simulink model "SP_OEL"  (R2023b)
settings: Solver=VariableStepAuto  StartTime=0.0  StopTime=1  RelTol=1e-3
undefined symbols (not defined in the file or in its folder): relay1, relay2, source
libraries: ee_lib x31, fl_lib x16, eeGeneralControl x8, nesl_utility x7, simulink x4, simulink_extras x4, spspowerguiLib x1
(part 1 of 2)
settings Model: Creator=hazwani  LastModifiedBy=yeowy
settings ModelReferenceCC: EnableRefExpFcnMdlSchedulingChecks=on

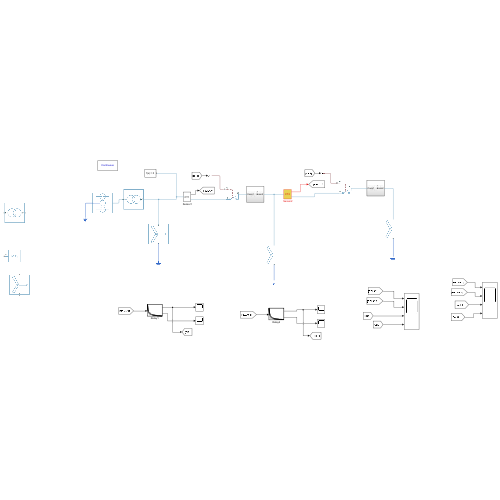
[thumbnail: Simulink's stored preview of the top-level diagram]
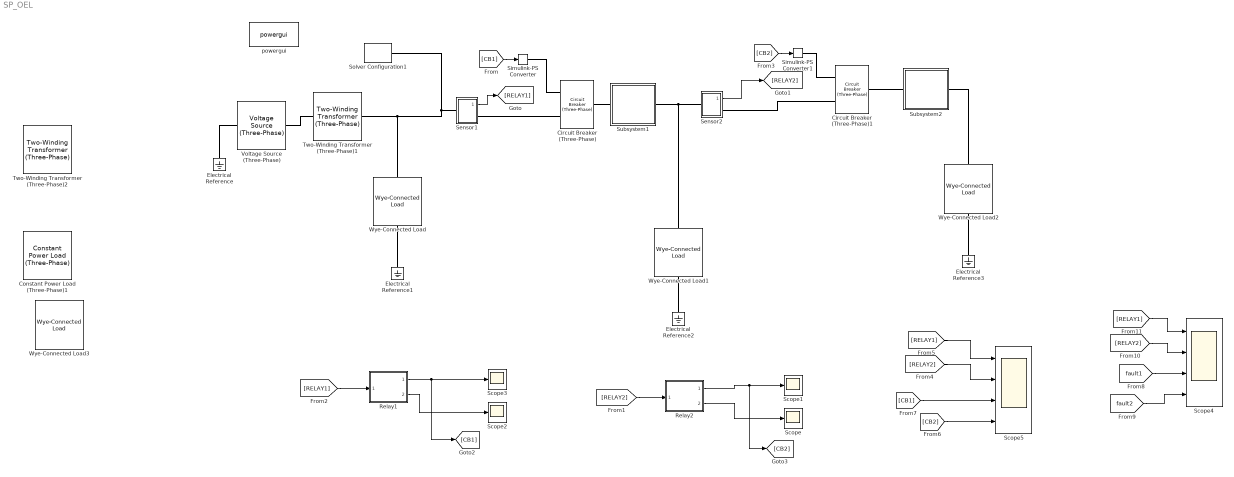
== system SP_OEL ==
  " Sensor1" : Subsystem
      mask Display: disp('CT1')
  " Sensor2" : Subsystem
      mask Display: disp('CT2')
  Circuit Breaker (Three-Phase) : ee_lib/Switches & Breakers/Circuit Breaker (Three-Phase)  R_closed=0.001 Ohm  G_open=1e-6 1/Ohm  threshold=11*(1./sqrt(3)) kV  breaker_behavior=ee.enum.switches.breakerBehavior.zeroCrossingEnable
      settings: InternalSimscapePortConfiguration="{\"Bottom\":[],\"Left\":[{\"id\":\"vT\",\"label\":\"vT\",\"type\":\"input\"},{\"id\":\"N1\",\"label\":\"~1\",\"type\":\"foundation.electrical.three_phase\"}],\"Right\":[{\"id\":\"N2\",\"label\":\"~2\",\"type\":\"foundation.electrical.three_phase\"}],\"Top\":[]}"
  Circuit Breaker (Three-Phase)1 : ee_lib/Switches & Breakers/Circuit Breaker (Three-Phase)  R_closed=0.001 Ohm  G_open=1e-6 1/Ohm  threshold=11*(1./sqrt(3)) kV  breaker_behavior=ee.enum.switches.breakerBehavior.zeroCrossingEnable
      settings: InternalSimscapePortConfiguration="{\"Bottom\":[],\"Left\":[{\"id\":\"vT\",\"label\":\"vT\",\"type\":\"input\"},{\"id\":\"N1\",\"label\":\"~1\",\"type\":\"foundation.electrical.three_phase\"}],\"Right\":[{\"id\":\"N2\",\"label\":\"~2\",\"type\":\"foundation.electrical.three_phase\"}],\"Top\":[]}"
  Constant Power Load (Three-Phase)1 : ee_lib/Passive/Constant Power Load (Three-Phase)  port_option=ee.enum.threePhasePort.composite  FRated=50 Hz  active_power=10 MW  reactive_power=4000 A*kV  Vline_rms_min=11 kV  tau=0.01 s  Vline_rms_ini=11 kV  Vang_ini=0 deg  gmin=1e-6 S  enable_fault=simscape.enum.onoff.off  fault_action=simscape.enum.assert.action.none  t_fault=1 s  open_conductance=1e-4 S
      settings: InternalSimscapePortConfiguration="{\"Bottom\":[],\"Left\":[{\"id\":\"N\",\"label\":\"~\",\"type\":\"foundation.electrical.three_phase\"}],\"Right\":[],\"Top\":[]}"
  Electrical Reference{,1..3} (4 alike) : fl_lib/Electrical/Electrical Elements/Electrical Reference
  Relay1 : Subsystem  TreatAsAtomicUnit=on  SystemSampleTime=relay1.sampleTime  mask{relayCharacteristicPhase=IEC Normal Inverse, relayCharacteristicEarth=IEC Normal Inverse, ratedFrequency=source.ratedFrequency, sampleTime=relay1.sampleTime, protectionEnable=1, currentPhase=[1.5 2.5 3.5 4.5 5.5 6.5 7.5 8.5 9.5 10.5], tmsPhase=[0.1 0.2], topPhase=[0.64 1.29;0.29 0.58;0.21 0.43;0.18 0.36;0.16 0.32;0.15 0.29;0.14 0.27;0.13 0.26;0.12 0.25;0.12 0.24], currentEarth=[0.06 0.15 0.2 0.25 0.3 0.35 0.4 0.45 0.5 0.55], tmsEarth=[0.1 0.2], topEarth=[0.64 1.29;0.29 0.58;0.21 0.43;0.18 0.36;0.16 0.32;0.15 0.29;0.14 0.27;0.13 0.26;0.12 0.25;0.12 0.24], phPickUp=relay1.phFltPickUp, ethPickUp=relay1.erFltPickUp, phTimeSetting=relay1.phFltTMS, ethTimeSetting=relay1.erFltTMS, topPhaseActual=0.2, topEarthActual=0.3}
      mask prompts: relayCharacteristicPhase "Relay characteristics for phase protection"; relayCharacteristicEarth "Relay characteristics for earth protection"; ratedFrequency "Fundamental frequency (Hz)"; sampleTime "Relay sample time (s)"; protectionEnable "Relay operation enable"; currentPhase "Current setting for phase protection (A)"; tmsPhase "Time multiplier setting for phase protection (s)"; topPhase "Operating time for phase protection (s)"; currentEarth "Current setting for earth protection (A)"; tmsEarth "Time multiplier setting for earth protection (s)"; topEarth "Operating time for earth protection (s)"; phPickUp "Pick up current for phase protection (A)"; ethPickUp "Pick up current for earth protection (A)"; phTimeSetting "Time multiplier setting for phase protection (s)"; ethTimeSetting "Time multiplier setting for earth protection (s)"; topPhaseActual "Relay operating time for phase protection (s)"; topEarthActual "Relay operating time for earth protection (s)"
      mask TypeOptions relayCharacteristicPhase: IEC Normal Inverse | IEC Very Inverse | IEC Extremely Inverse | IEEE Moderately Inverse | IEEE Very Inverse | IEEE Extremely Inverse | Definite Time | IvsT
      mask Callback relayCharacteristicPhase:
      | % Control parameter visiblity
      | enablePhase = get_param(gcb,'relayCharacteristicPhase');
      | enableEarth = get_param(gcb,'relayCharacteristicEarth');
      | % Set the 'MaskVisibilities' property for each parameters
      | cArray=cell(1,17);
      | cArray(:)={'on'};
      | p=strcmp(enablePhase,'IvsT');
      | q=strcmp(enableEarth,'IvsT');
      | r=strcmp(enablePhase,'Definite Time');
      | s=strcmp(enableEarth,'Definite Time');
      | if p==0 && q==1
      |     cArray(6:8)={'off'};
      | elseif p==0 && q==0
      |     cArray(6:11)={'off'};
      | elseif p==1 && q==0
      |     cArray(9:11)={'off'};
      | end
      | if r==0 && s==1
      |     cArray(15)={'off'};
      |     cArray(16)={'off'};
      | elseif r==0 && s==0
      |     cArray(16:17)={'off'};
      | elseif r==1 && s==0
      |     cArray(14)={'off'};
      |     cArray(17)={'off'};
      | elseif r==1 && s==1
      |     cArray(14:15)={'off'};
      | end
      | set_param(gcb,'MaskVisibilities',cArray);
      mask TypeOptions relayCharacteristicEarth: IEC Normal Inverse | IEC Very Inverse | IEC Extremely Inverse | IEEE Moderately Inverse | IEEE Very Inverse | IEEE Extremely Inverse | Definite Time | IvsT
      mask Callback relayCharacteristicEarth:
      | % Control parameter visiblity
      | enablePhase = get_param(gcb,'relayCharacteristicPhase');
      | enableEarth = get_param(gcb,'relayCharacteristicEarth');
      | % Set the 'MaskVisibilities' property for each parameters
      | cArray=cell(1,17);
      | cArray(:)={'on'};
      | p=strcmp(enablePhase,'IvsT');
      | q=strcmp(enableEarth,'IvsT');
      | r=strcmp(enablePhase,'Definite Time');
      | s=strcmp(enableEarth,'Definite Time');
      | if p==0 && q==1
      |     cArray(6:8)={'off'};
      | elseif p==0 && q==0
      |     cArray(6:11)={'off'};
      | elseif p==1 && q==0
      |     cArray(9:11)={'off'};
      | end
      | if r==0 && s==1
      |     cArray(15)={'off'};
      |     cArray(16)={'off'};
      | elseif r==0 && s==0
      |     cArray(16:17)={'off'};
      | elseif r==1 && s==0
      |     cArray(14)={'off'};
      |     cArray(17)={'off'};
      | elseif r==1 && s==1
      |     cArray(14:15)={'off'};
      | end
      | set_param(gcb,'MaskVisibilities',cArray);
      mask DialogControl Container9 Prompt: Main
      mask DialogControl Container24 Prompt: Current Settings
      mask DialogControl Container19 Prompt: Time Settings
      mask Display:
      | psm = 1:1:30; % Plug setting multiplier
      | tms=0.01; % Time multiplier setting is assumed to be 0.01s
      | top=ones(2,length(psm));  % Operating time of the relay
      | maskParameter=Simulink.Mask.get(gcb); % Get the mask parameters
      | for i=1:2
      |     index(i)=find(strcmp(maskParameter.Parameters(1,i).Value,maskParameter.Parameters(1,i).TypeOptions));
      |     if index(i)<7
      |         switch index(i)              % Selection of relay characteristic
      |             case 1                   % IEC Normal Inverse
      |                 a=0.14;
      |                 b=0.02;
      |                 c=0;
      |             case 2                   % IEC Very Inverse
      |                 a=13.5;
      |                 b=1;
      |                 c=0;
      |             case 3                   % IEC Extremely Inverse
      |                 a=80;
      |                 b=2;
      |                 c=0;
      |             case 4                   % IEEE Moderately Inverse
      |                 a=0.0515;
      |                 b=0.02;
      |                 c=0.114;
      |             case 5                   % IEEE Very Inverse
      |                 a=19.61;
      |                 b=2;
      |                 c=0.491;
      |             otherwise                % IEEE Exteremely Inverse
      |                 a=28.2;
      |                 b=2;
      |                 c=0.1217;
      |         end
      |         for j=1:length(psm)
      |             top(i,j)=tms*((a/(power(psm(j),b)-1))+c); % Operating time of the relay
      |         end
      |     else
      |         top(i,1:length(psm))=0.03*ones(1,length(psm));% Operating time of the relay
      |     end
      | end
      | top1=top(1,1:end);
      | top2=top(2,1:end);
      | 
      | maskFigure=figure;
      | if index(1)<8
      |     plot(psm,top1)
      | else
      |     fprintf('\n\nIvsT');
      | end
      | hold on;
      | if index(2)<8
      |     plot(psm,top2);
      | elseif index(1)<8
      |     fprintf('\nIvsT');
      | end
      | close(maskFigure);
  Relay2 : Subsystem  TreatAsAtomicUnit=on  SystemSampleTime=relay1.sampleTime  mask{relayCharacteristicPhase=IEEE Moderately Inverse, relayCharacteristicEarth=IEEE Moderately Inverse, ratedFrequency=source.ratedFrequency, sampleTime=relay2.sampleTime, protectionEnable=1, currentPhase=[1.5 2.5 3.5 4.5 5.5 6.5 7.5 8.5 9.5 10.5], tmsPhase=[0.1 0.2], topPhase=[0.64 1.29;0.29 0.58;0.21 0.43;0.18 0.36;0.16 0.32;0.15 0.29;0.14 0.27;0.13 0.26;0.12 0.25;0.12 0.24], currentEarth=[0.06 0.15 0.2 0.25 0.3 0.35 0.4 0.45 0.5 0.55], tmsEarth=[0.1 0.2], topEarth=[0.64 1.29;0.29 0.58;0.21 0.43;0.18 0.36;0.16 0.32;0.15 0.29;0.14 0.27;0.13 0.26;0.12 0.25;0.12 0.24], phPickUp=relay2.phFltPickUp, ethPickUp=relay2.erFltPickUp, phTimeSetting=relay2.phFltTMS, ethTimeSetting=relay2.erFltTMS, topPhaseActual=0.2, topEarthActual=0.3}
      mask prompts: relayCharacteristicPhase "Relay characteristics for phase protection"; relayCharacteristicEarth "Relay characteristics for earth protection"; ratedFrequency "Fundamental frequency (Hz)"; sampleTime "Relay sample time (s)"; protectionEnable "Relay operation enable"; currentPhase "Current setting for phase protection (A)"; tmsPhase "Time multiplier setting for phase protection (s)"; topPhase "Operating time for phase protection (s)"; currentEarth "Current setting for earth protection (A)"; tmsEarth "Time multiplier setting for earth protection (s)"; topEarth "Operating time for earth protection (s)"; phPickUp "Pick up current for phase protection (A)"; ethPickUp "Pick up current for earth protection (A)"; phTimeSetting "Time multiplier setting for phase protection (s)"; ethTimeSetting "Time multiplier setting for earth protection (s)"; topPhaseActual "Relay operating time for phase protection (s)"; topEarthActual "Relay operating time for earth protection (s)"
      mask TypeOptions relayCharacteristicPhase: IEC Normal Inverse | IEC Very Inverse | IEC Extremely Inverse | IEEE Moderately Inverse | IEEE Very Inverse | IEEE Extremely Inverse | Definite Time | IvsT
      mask Callback relayCharacteristicPhase:
      | % Control parameter visiblity
      | enablePhase = get_param(gcb,'relayCharacteristicPhase');
      | enableEarth = get_param(gcb,'relayCharacteristicEarth');
      | % Set the 'MaskVisibilities' property for each parameters
      | cArray=cell(1,17);
      | cArray(:)={'on'};
      | p=strcmp(enablePhase,'IvsT');
      | q=strcmp(enableEarth,'IvsT');
      | r=strcmp(enablePhase,'Definite Time');
      | s=strcmp(enableEarth,'Definite Time');
      | if p==0 && q==1
      |     cArray(6:8)={'off'};
      | elseif p==0 && q==0
      |     cArray(6:11)={'off'};
      | elseif p==1 && q==0
      |     cArray(9:11)={'off'};
      | end
      | if r==0 && s==1
      |     cArray(15)={'off'};
      |     cArray(16)={'off'};
      | elseif r==0 && s==0
      |     cArray(16:17)={'off'};
      | elseif r==1 && s==0
      |     cArray(14)={'off'};
      |     cArray(17)={'off'};
      | elseif r==1 && s==1
      |     cArray(14:15)={'off'};
      | end
      | set_param(gcb,'MaskVisibilities',cArray);
      mask TypeOptions relayCharacteristicEarth: IEC Normal Inverse | IEC Very Inverse | IEC Extremely Inverse | IEEE Moderately Inverse | IEEE Very Inverse | IEEE Extremely Inverse | Definite Time | IvsT
      mask Callback relayCharacteristicEarth:
      | % Control parameter visiblity
      | enablePhase = get_param(gcb,'relayCharacteristicPhase');
      | enableEarth = get_param(gcb,'relayCharacteristicEarth');
      | % Set the 'MaskVisibilities' property for each parameters
      | cArray=cell(1,17);
      | cArray(:)={'on'};
      | p=strcmp(enablePhase,'IvsT');
      | q=strcmp(enableEarth,'IvsT');
      | r=strcmp(enablePhase,'Definite Time');
      | s=strcmp(enableEarth,'Definite Time');
      | if p==0 && q==1
      |     cArray(6:8)={'off'};
      | elseif p==0 && q==0
      |     cArray(6:11)={'off'};
      | elseif p==1 && q==0
      |     cArray(9:11)={'off'};
      | end
      | if r==0 && s==1
      |     cArray(15)={'off'};
      |     cArray(16)={'off'};
      | elseif r==0 && s==0
      |     cArray(16:17)={'off'};
      | elseif r==1 && s==0
      |     cArray(14)={'off'};
      |     cArray(17)={'off'};
      | elseif r==1 && s==1
      |     cArray(14:15)={'off'};
      | end
      | set_param(gcb,'MaskVisibilities',cArray);
      mask DialogControl Container9 Prompt: Main
      mask DialogControl Container24 Prompt: Current Settings
      mask DialogControl Container19 Prompt: Time Settings
      mask Display:
      | psm = 1:1:30; % Plug setting multiplier
      | tms=0.01; % Time multiplier setting is assumed to be 0.01s
      | top=ones(2,length(psm));  % Operating time of the relay
      | maskParameter=Simulink.Mask.get(gcb); % Get the mask parameters
      | for i=1:2
      |     index(i)=find(strcmp(maskParameter.Parameters(1,i).Value,maskParameter.Parameters(1,i).TypeOptions));
      |     if index(i)<7
      |         switch index(i)              % Selection of relay characteristic
      |             case 1                   % IEC Normal Inverse
      |                 a=0.14;
      |                 b=0.02;
      |                 c=0;
      |             case 2                   % IEC Very Inverse
      |                 a=13.5;
      |                 b=1;
      |                 c=0;
      |             case 3                   % IEC Extremely Inverse
      |                 a=80;
      |                 b=2;
      |                 c=0;
      |             case 4                   % IEEE Moderately Inverse
      |                 a=0.0515;
      |                 b=0.02;
      |                 c=0.114;
      |             case 5                   % IEEE Very Inverse
      |                 a=19.61;
      |                 b=2;
      |                 c=0.491;
      |             otherwise                % IEEE Exteremely Inverse
      |                 a=28.2;
      |                 b=2;
      |                 c=0.1217;
      |         end
      |         for j=1:length(psm)
      |             top(i,j)=tms*((a/(power(psm(j),b)-1))+c); % Operating time of the relay
      |         end
      |     else
      |         top(i,1:length(psm))=0.03*ones(1,length(psm));% Operating time of the relay
      |     end
      | end
      | top1=top(1,1:end);
      | top2=top(2,1:end);
      | 
      | maskFigure=figure;
      | if index(1)<8
      |     plot(psm,top1)
      | else
      |     fprintf('\n\nIvsT');
      | end
      | hold on;
      | if index(2)<8
      |     plot(psm,top2);
      | elseif index(1)<8
      |     fprintf('\nIvsT');
      | end
      | close(maskFigure);
  Scope{,1..3} (4 alike) : Scope
  Scope4 : Scope  NumInputPorts=4
  Scope5 : Scope  NumInputPorts=4
  Simulink-PS Converter : nesl_utility/Simulink-PS Converter  PhysicalDomain=network_engine_domain  SubClassName=ps_input  LeftPortType=input  RightPortType=output  PseudoPeriodic=off  Frequencies=[]  NoiseDistribution=none  NoiseParameters=[]  Unit=1  AffineConversion=off  FilteringAndDerivatives=provide  SimscapeFilterOrder=1  InputFilterTimeConstant=0.001  UdotUserProvided=0
  Simulink-PS Converter1 : nesl_utility/Simulink-PS Converter  PhysicalDomain=network_engine_domain  SubClassName=ps_input  LeftPortType=input  RightPortType=output  PseudoPeriodic=off  Frequencies=[]  NoiseDistribution=none  NoiseParameters=[]  Unit=1  AffineConversion=off  FilteringAndDerivatives=provide  SimscapeFilterOrder=1  InputFilterTimeConstant=0.001  UdotUserProvided=0
  Solver Configuration1 : nesl_utility/Solver Configuration  PhysicalDomain=network_engine_domain  SubClassName=solver  LeftPortType=input  RightPortType=generic  Tones=[]  Harmonics=[]  SimulateNoise=off  Profile=off  UseLocalSampling=off  EnableSwitchedLinearOptims=on  FrequencyDomain=off  UseCCode=off  RelTol=0.001  AbsTol=0.001  MinStep=1e-09  ToWorkspace=off  RevertToSquareIcSolve=off  NumHomotopyIterations=100  PhasorMode=off  PhasorModeNumHarmonics=1  ConsistencySolver=NEWTON_XTOL_AFTER_FTOL  IndexReductionMethod=DerivativeReplacement  DoDC=on  ResidualTolerance=1e-09  ConsistencyTolSource=LOCAL  ConsistencyAbsTol=0.001  ConsistencyRelTol=0.001  ConsistencyTolFactor=0.001  UseLocalSolver=on  LocalSolverChoice=NE_TRAPEZOIDAL_ADVANCER  ResolveIndetEquations=on  FunctionEvalNumThread=1  LocalSolverSampleTime=0.001  DoFixedCost=on  MaxNonlinIter=3  MaxModeIter=2  ComputeImpulses=off  ImpulseIterations=2  LinearAlgebra=auto  LinearAlgebraNumThread=0  EquationFormulation=NE_TIME_EF  DelaysMemoryBudget=1024  AutomaticFiltering=on  FilteringTimeConstant=0.001  PartitionStorageMethod=AS_NEEDED  PartitionMemoryBudget=1024  PartitionMethod=ROBUST  MultibodyUseLocalSolver=off  MultibodyLocalSolverChoice=ODE1  MultibodyLocalSolverSampleTime=0.001
  Subsystem1 : Subsystem
  Subsystem2 : Subsystem
  Two-Winding Transformer (Three-Phase)1 : ee_lib/Passive/Transformers/Two-Winding Transformer (Three-Phase)  SRated=60e6 A*V  FRated=50 Hz  Winding1Connection=ee.enum.windingconnection.delta1  VRated1=33*(1./sqrt(3)) kV  Winding2Connection=ee.enum.windingconnection.Y  VRated2=11*(1./sqrt(3)) kV  CoreType=ee.enum.coretype.fivelimb  pu_Rw1=0.0014  pu_Rw2=0.0014  leakage_reactance_option=ee.enum.transformer_leakage.include  pu_Xl1=0.0624  pu_Xl2=0.0624  magnetizing_resistance_option=ee.enum.transformer_magnetizingResistance.include  pu_Rm=450  magnetizing_reactance_option=ee.enum.transformer_magnetizingReactance.include  saturation_option=ee.enum.transformer_saturation.exclude  pu_Xm=450  current_data=[0, .002, 1, 2]  magnetic_flux_data=[0, 1.2, 1.5, 1.51]  pu_X0=0.5  i1_specify=off  i1_priority=None  i1=[0, 0, 0] A  i1_nominal_specify=off  i1_nominal_unit=A  i1_nominal_value=1  i2_specify=off  i2_priority=None  i2=[0, 0, 0] A  i2_nominal_specify=off  i2_nominal_unit=A  i2_nominal_value=1  phi_specify=off  phi_priority=None  phi=[0, 0, 0]  phi_nominal_specify=off  phi_nominal_unit=1  phi_nominal_value=1  power_dissipated_specify=off  power_dissipated_priority=None  power_dissipated=0 W  power_dissipated_nominal_specify=off  power_dissipated_nominal_unit=W  power_dissipated_nominal_value=1
      settings: InternalSimscapePortConfiguration="{\"Bottom\":[],\"Left\":[{\"id\":\"N1\",\"label\":\"~1\",\"type\":\"foundation.electrical.three_phase\"}],\"Right\":[{\"id\":\"N2\",\"label\":\"~2\",\"type\":\"foundation.electrical.three_phase\"}],\"Top\":[]}"
  Two-Winding Transformer (Three-Phase)2 : ee_lib/Passive/Transformers/Two-Winding Transformer (Three-Phase)  SRated=60e6 A*V  FRated=50 Hz  Winding1Connection=ee.enum.windingconnection.delta1  VRated1=33*(1./sqrt(3)) kV  Winding2Connection=ee.enum.windingconnection.Y  VRated2=11*(1./sqrt(3)) kV  CoreType=ee.enum.coretype.fivelimb  pu_Rw1=0.0014  pu_Rw2=0.0014  leakage_reactance_option=ee.enum.transformer_leakage.include  pu_Xl1=0.0624  pu_Xl2=0.0624  magnetizing_resistance_option=ee.enum.transformer_magnetizingResistance.include  pu_Rm=450  magnetizing_reactance_option=ee.enum.transformer_magnetizingReactance.include  saturation_option=ee.enum.transformer_saturation.exclude  pu_Xm=450  current_data=[0, .002, 1, 2]  magnetic_flux_data=[0, 1.2, 1.5, 1.51]  pu_X0=0.5  i1_specify=off  i1_priority=None  i1=[0, 0, 0] A  i1_nominal_specify=off  i1_nominal_unit=A  i1_nominal_value=1  i2_specify=off  i2_priority=None  i2=[0, 0, 0] A  i2_nominal_specify=off  i2_nominal_unit=A  i2_nominal_value=1  phi_specify=off  phi_priority=None  phi=[0, 0, 0]  phi_nominal_specify=off  phi_nominal_unit=1  phi_nominal_value=1  power_dissipated_specify=off  power_dissipated_priority=None  power_dissipated=0 W  power_dissipated_nominal_specify=off  power_dissipated_nominal_unit=W  power_dissipated_nominal_value=1
      settings: InternalSimscapePortConfiguration="{\"Bottom\":[],\"Left\":[{\"id\":\"N1\",\"label\":\"~1\",\"type\":\"foundation.electrical.three_phase\"}],\"Right\":[{\"id\":\"N2\",\"label\":\"~2\",\"type\":\"foundation.electrical.three_phase\"}],\"Top\":[]}"
  Voltage Source (Three-Phase) : ee_lib/Sources/Voltage Source (Three-Phase)  vline_rms=33*(1./sqrt(3)) kV  shift=0 deg  freq=50 Hz  impedance_option=1  SShortCircuit=800e6 A*V  XR=5  R=0.01 Ohm  L=3.97e-4 H  harmonic_option=0  harmonic_orders=[5, 7, 11, 13]  harmonic_ratios=[.1, .1, .1, .1]  G_parasitic=0 1/Ohm  I_specify=off  I_priority=None  I=[0, 0, 0] A  I_nominal_specify=off  I_nominal_unit=A  I_nominal_value=1
  Wye-Connected Load : ee_lib/Passive/RLC Assemblies/Wye-Connected Load  parameterization=ee.enum.rlc.parameterization.ratedpower  component_structure=ee.enum.rlc.structure.R  component_structure_PQ=ee.enum.rlc.structure.SeriesRL  R=1 Ohm  L=1e-3 H  C=1e-6 F  VRated=11*(1./sqrt(3)) kV  FRated=50 Hz  P=10 MW  Qpos=4e6 A*V  Qneg=-1e2 A*V  R_parasitic=0 Ohm  G_parasitic=0 1/Ohm  R_parasitic_PQ=0 Ohm  G_parasitic_PQ=1e-6 1/Ohm  Vmag0=11*(1./sqrt(3)) kV  Vang0=0 deg  Freq0=50 Hz  IL_specify=off  IL_priority=High  IL=[0, 0, 0] A  IL_nominal_specify=off  IL_nominal_unit=A  IL_nominal_value=1  VC_specify=off  VC_priority=High  VC=[0, 0, 0] V  VC_nominal_specify=off  VC_nominal_unit=V  VC_nominal_value=1
  Wye-Connected Load1 : ee_lib/Passive/RLC Assemblies/Wye-Connected Load  parameterization=ee.enum.rlc.parameterization.ratedpower  component_structure=ee.enum.rlc.structure.R  component_structure_PQ=ee.enum.rlc.structure.SeriesRL  R=1 Ohm  L=1e-3 H  C=1e-6 F  VRated=11*(1./sqrt(3)) kV  FRated=50 Hz  P=10 MW  Qpos=4e6 A*V  Qneg=-1e2 A*V  R_parasitic=0 Ohm  G_parasitic=0 1/Ohm  R_parasitic_PQ=0 Ohm  G_parasitic_PQ=1e-6 1/Ohm  Vmag0=11*(1./sqrt(3)) kV  Vang0=0 deg  Freq0=50 Hz  IL_specify=off  IL_priority=High  IL=[0, 0, 0] A  IL_nominal_specify=off  IL_nominal_unit=A  IL_nominal_value=1  VC_specify=off  VC_priority=High  VC=[0, 0, 0] V  VC_nominal_specify=off  VC_nominal_unit=V  VC_nominal_value=1
  Wye-Connected Load2 : ee_lib/Passive/RLC Assemblies/Wye-Connected Load  parameterization=ee.enum.rlc.parameterization.ratedpower  component_structure=ee.enum.rlc.structure.R  component_structure_PQ=ee.enum.rlc.structure.SeriesRL  R=1 Ohm  L=1e-3 H  C=1e-6 F  VRated=11*(1./sqrt(3)) kV  FRated=50 Hz  P=20 MW  Qpos=10e6 A*V  Qneg=-1e2 A*V  R_parasitic=0 Ohm  G_parasitic=0 1/Ohm  R_parasitic_PQ=0 Ohm  G_parasitic_PQ=1e-6 1/Ohm  Vmag0=11*(1./sqrt(3)) kV  Vang0=0 deg  Freq0=50 Hz  IL_specify=off  IL_priority=High  IL=[0, 0, 0] A  IL_nominal_specify=off  IL_nominal_unit=A  IL_nominal_value=1  VC_specify=off  VC_priority=High  VC=[0, 0, 0] V  VC_nominal_specify=off  VC_nominal_unit=V  VC_nominal_value=1
  Wye-Connected Load3 : ee_lib/Passive/RLC Assemblies/Wye-Connected Load  parameterization=ee.enum.rlc.parameterization.ratedpower  component_structure=ee.enum.rlc.structure.R  component_structure_PQ=ee.enum.rlc.structure.SeriesRL  R=1 Ohm  L=1e-3 H  C=1e-6 F  VRated=11*(1./sqrt(3)) kV  FRated=50 Hz  P=10 MW  Qpos=4e6 A*V  Qneg=-1e2 A*V  R_parasitic=0 Ohm  G_parasitic=0 1/Ohm  R_parasitic_PQ=0 Ohm  G_parasitic_PQ=1e-6 1/Ohm  Vmag0=24e3 V  Vang0=0 deg  Freq0=60 Hz  IL_specify=off  IL_priority=High  IL=[0, 0, 0] A  IL_nominal_specify=off  IL_nominal_unit=A  IL_nominal_value=1  VC_specify=off  VC_priority=High  VC=[0, 0, 0] V  VC_nominal_specify=off  VC_nominal_unit=V  VC_nominal_value=1
  powergui : spspowerguiLib/powergui  Priority=1  SimulationMode=Continuous  SampleTime=50e-6  frequency=60  Iterations=50  frequencyindice=60  Pbase=100e6  ErrMax=1e-4  UnitsV=kV  UnitsW=MW  buscounter=0  FunctionMessages=off  echomessages=off  EnableUseOfTLC=off  CurrentSourceSwitches=off  DisableSnubberDevices=off  DisableRonSwitches=off  DisableVfSwitches=off  DisplayEquations=off  AutomaticDiscreteSolvers=off  SolverType=Tustin/Backward Euler (TBE)  Interpol=off  ExternalGateDelay=off  methode=off  Ts=100  x0status=blocks  SPID=on  SwTol=0  HookPort=off  NonlinearTolerance=1e-4  nMaxIteration=100  ContinueOnMaxIteration=off  RestoreLinks=warning  ResistiveCurrentMeasurement=off  Frange=[0:2:500]  Ylog=off  Xlog=on  ShowGrid=off  save=off  variable=ZData  structure=0  ZoomFFT=off  StartTime=0.0  cycles=1  DisplayStyle=1  fundamental=60  FreqAxis=off  MaxFrequency=1000  frequencyindicesteady=1  RmsSteady=1  display=off
  wires:
  " Sensor1"/1(Out1) -> [RELAY1]
  Relay2/2(Relay Status) -> Scope/1
  Relay2/1(Trip Signal) -> [CB2], Scope1/1
  Relay1/1(Trip Signal) -> [CB1], Scope3/1
  " Sensor2"/1(Out1) -> [RELAY2]
  [CB1] -> Simulink-PS Converter/1
  [CB2] -> Simulink-PS Converter1/1
  [RELAY2] -> Relay2/1(Inport)
  [RELAY1] -> Relay1/1(Inport)
  Relay1/2(Relay Status) -> Scope2/1
  [RELAY2] -> Scope5/2
  [RELAY1] -> Scope5/1
  [CB1] -> Scope5/3
  [CB2] -> Scope5/4
  [RELAY1] -> Scope4/1
  [RELAY2] -> Scope4/2
  [fault1] -> Scope4/3
  [fault2] -> Scope4/4
  connections:
  Voltage Source (Three-Phase)/LConn1 -- Electrical Reference/LConn1
  Two-Winding Transformer (Three-Phase)1/LConn1 -- Voltage Source (Three-Phase)/RConn1
  Electrical Reference1/LConn1 -- Wye-Connected Load/RConn1
  Solver Configuration1/RConn1 -- Two-Winding Transformer (Three-Phase)1/RConn1 -- Wye-Connected Load/LConn1 -- " Sensor1"/LConn1
  " Sensor1"/RConn1 -- Circuit Breaker (Three-Phase)/LConn2
  Circuit Breaker (Three-Phase)/RConn1 -- Subsystem1/LConn1
  Simulink-PS Converter/RConn1 -- Circuit Breaker (Three-Phase)/LConn1
  Circuit Breaker (Three-Phase)1/LConn1 -- Simulink-PS Converter1/RConn1
  Circuit Breaker (Three-Phase)1/RConn1 -- Subsystem2/LConn1
  Subsystem1/RConn1 -- Wye-Connected Load1/LConn1 -- " Sensor2"/LConn1
  Circuit Breaker (Three-Phase)1/LConn2 -- " Sensor2"/RConn1
  Wye-Connected Load1/RConn1 -- Electrical Reference2/LConn1
  Electrical Reference3/LConn1 -- Wye-Connected Load2/RConn1
  Wye-Connected Load2/LConn1 -- Subsystem2/RConn1

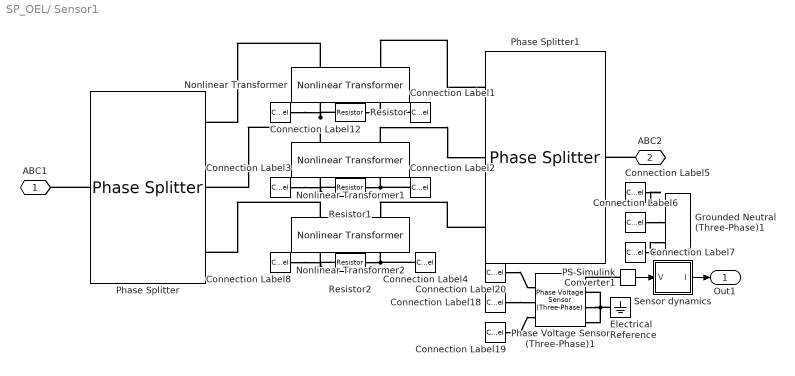
== system SP_OEL/ Sensor1 ==
  Connection Label1 : ConnectionLabel  Label=Ian
  Connection Label12 : ConnectionLabel  Label=Iap
  Connection Label18 : ConnectionLabel  Label=Ibp
  Connection Label19 : ConnectionLabel  Label=Icp
  Connection Label2 : ConnectionLabel  Label=Ibn
  Connection Label20 : ConnectionLabel  Label=Iap
  Connection Label3 : ConnectionLabel  Label=Ibp
  Connection Label4 : ConnectionLabel  Label=Ibn
  Connection Label5 : ConnectionLabel  Label=Ian
  Connection Label6 : ConnectionLabel  Label=Ibn
  Connection Label7 : ConnectionLabel  Label=Icn
  Connection Label8 : ConnectionLabel  Label=Icp
  Electrical Reference : fl_lib/Electrical/Electrical Elements/Electrical Reference
  Grounded Neutral (Three-Phase)1 : ee_lib/Connectors & References/Grounded Neutral (Three-Phase)
      settings: InternalSimscapePortConfiguration="{\"Bottom\":[],\"Left\":[{\"id\":\"a\",\"label\":\"a\",\"type\":\"foundation.electrical.electrical\"},{\"id\":\"b\",\"label\":\"b\",\"type\":\"foundation.electrical.electrical\"},{\"id\":\"c\",\"label\":\"c\",\"type\":\"foundation.electrical.electrical\"}],\"Right\":[],\"Top\":[]}"
  Nonlinear Transformer : ee_lib/Passive/Transformers/Nonlinear Transformer  Nw=1  Nw2=sensor1.ctRatio  winding_param_option=1  Req=1e-3 Ohm  Leq=1e-4 H  R_1=0.01 Ohm  L_1=0.0001 H  R_2=0.01 Ohm  L_2=0.0001 H  averaging_period=0 s  R_m=100 Ohm  parameterization_option=1  H_data=[0, 200, 400, 600, 800, 1000] A/m  B_data=[0, .81, 1.25, 1.42, 1.48, 1.49] T  length_effective=0.2 m  area_effective=2e-4 m^2  L=4e-2 H  L_sat=1e-2 H  current_data=[0, .4, .8, 1.2, 1.6, 2] A  magnetic_flux_data=[0, .161, .25, .284, .295, .299] .* 1e-3 Wb  magnetic_flux_sat=1.6e-04 Wb  dBdH0=0.005 m*T/A  B1=1.49 T  H1=1000 A/m  c=0.1  K=200 A/m  alpha=1e-4  interpolation_option=1  Leq_i0=0 A  L1_i0=0 A  L2_i0=0 A  x0_option=1  i_L0=0 A  phi0=0 Wb  B0=0 T  H0=0 A/m  Leq_g=1e-9 1/Ohm  L1_g=1e-9 1/Ohm  L2_g=1e-9 1/Ohm
      settings: InternalSimscapePortConfiguration="{\"Bottom\":[],\"Left\":[{\"id\":\"p1\",\"label\":\"1+\",\"type\":\"foundation.electrical.electrical\"},{\"id\":\"n1\",\"label\":\"1-\",\"type\":\"foundation.electrical.electrical\"}],\"Right\":[{\"id\":\"p2\",\"label\":\"2+\",\"type\":\"foundation.electrical.electrical\"},{\"id\":\"n2\",\"label\":\"2-\",\"type\":\"foundation.electrical.electrical\"}],\"Top\":[]}"
  Nonlinear Transformer1 : ee_lib/Passive/Transformers/Nonlinear Transformer  Nw=1  Nw2=sensor1.ctRatio  winding_param_option=1  Req=1e-3 Ohm  Leq=1e-4 H  R_1=0.01 Ohm  L_1=0.0001 H  R_2=0.01 Ohm  L_2=0.0001 H  averaging_period=0 s  R_m=100 Ohm  parameterization_option=1  H_data=[0, 200, 400, 600, 800, 1000] A/m  B_data=[0, .81, 1.25, 1.42, 1.48, 1.49] T  length_effective=0.2 m  area_effective=2e-4 m^2  L=4e-2 H  L_sat=1e-2 H  current_data=[0, .4, .8, 1.2, 1.6, 2] A  magnetic_flux_data=[0, .161, .25, .284, .295, .299] .* 1e-3 Wb  magnetic_flux_sat=1.6e-04 Wb  dBdH0=0.005 m*T/A  B1=1.49 T  H1=1000 A/m  c=0.1  K=200 A/m  alpha=1e-4  interpolation_option=1  Leq_i0=0 A  L1_i0=0 A  L2_i0=0 A  x0_option=1  i_L0=0 A  phi0=0 Wb  B0=0 T  H0=0 A/m  Leq_g=1e-9 1/Ohm  L1_g=1e-9 1/Ohm  L2_g=1e-9 1/Ohm
      settings: InternalSimscapePortConfiguration="{\"Bottom\":[],\"Left\":[{\"id\":\"p1\",\"label\":\"1+\",\"type\":\"foundation.electrical.electrical\"},{\"id\":\"n1\",\"label\":\"1-\",\"type\":\"foundation.electrical.electrical\"}],\"Right\":[{\"id\":\"p2\",\"label\":\"2+\",\"type\":\"foundation.electrical.electrical\"},{\"id\":\"n2\",\"label\":\"2-\",\"type\":\"foundation.electrical.electrical\"}],\"Top\":[]}"
  Nonlinear Transformer2 : ee_lib/Passive/Transformers/Nonlinear Transformer  Nw=1  Nw2=sensor1.ctRatio  winding_param_option=1  Req=1e-3 Ohm  Leq=1e-4 H  R_1=0.01 Ohm  L_1=0.0001 H  R_2=0.01 Ohm  L_2=0.0001 H  averaging_period=0 s  R_m=100 Ohm  parameterization_option=1  H_data=[0, 200, 400, 600, 800, 1000] A/m  B_data=[0, .81, 1.25, 1.42, 1.48, 1.49] T  length_effective=0.2 m  area_effective=2e-4 m^2  L=4e-2 H  L_sat=1e-2 H  current_data=[0, .4, .8, 1.2, 1.6, 2] A  magnetic_flux_data=[0, .161, .25, .284, .295, .299] .* 1e-3 Wb  magnetic_flux_sat=1.6e-04 Wb  dBdH0=0.005 m*T/A  B1=1.49 T  H1=1000 A/m  c=0.1  K=200 A/m  alpha=1e-4  interpolation_option=1  Leq_i0=0 A  L1_i0=0 A  L2_i0=0 A  x0_option=1  i_L0=0 A  phi0=0 Wb  B0=0 T  H0=0 A/m  Leq_g=1e-9 1/Ohm  L1_g=1e-9 1/Ohm  L2_g=1e-9 1/Ohm
      settings: InternalSimscapePortConfiguration="{\"Bottom\":[],\"Left\":[{\"id\":\"p1\",\"label\":\"1+\",\"type\":\"foundation.electrical.electrical\"},{\"id\":\"n1\",\"label\":\"1-\",\"type\":\"foundation.electrical.electrical\"}],\"Right\":[{\"id\":\"p2\",\"label\":\"2+\",\"type\":\"foundation.electrical.electrical\"},{\"id\":\"n2\",\"label\":\"2-\",\"type\":\"foundation.electrical.electrical\"}],\"Top\":[]}"
  PS-Simulink Converter1 : nesl_utility/PS-Simulink Converter  PhysicalDomain=network_engine_domain  SubClassName=ps_output  LeftPortType=input  RightPortType=output  PseudoPeriodic=off  Frequencies=[]  VectorFormat=1-D array  Unit=inherit  AffineConversion=off
  Phase Splitter : ee_lib/Connectors & References/Phase Splitter
  Phase Splitter1 : ee_lib/Connectors & References/Phase Splitter
  Phase Voltage Sensor (Three-Phase)1 : ee_lib/Sensors & Transducers/Phase Voltage Sensor (Three-Phase)
      settings: LogSimulationData=on  InternalSimscapePortConfiguration="{\"Bottom\":[],\"Left\":[{\"id\":\"a1\",\"label\":\"a1\",\"type\":\"foundation.electrical.electrical\"},{\"id\":\"b1\",\"label\":\"b1\",\"type\":\"foundation.electrical.electrical\"},{\"id\":\"c1\",\"label\":\"c1\",\"type\":\"foundation.electrical.electrical\"}],\"Right\":[{\"id\":\"V_output\",\"label\":\"V\",\"type\":\"output\"},{\"id\":\"a2\",\"label\":\"a2\",\"type\":\"foundation.electrical.electrical\"},{\"id\":\"b2\",\"label\":\"b2\",\"type\":\"foundation.electrical.electrical\"},{\"id\":\"c2\",\"label\":\"c2\",\"type\":\"foundation.electrical.electrical\"}],\"Top\":[]}"
  Resistor : fl_lib/Electrical/Electrical Elements/Resistor  R=1 Ohm  i_specify=off  i_priority=None  i=0 A  i_nominal_specify=off  i_nominal_unit=A  i_nominal_value=1  v_specify=off  v_priority=None  v=0 V  v_nominal_specify=off  v_nominal_unit=V  v_nominal_value=1
  Resistor1 : fl_lib/Electrical/Electrical Elements/Resistor  R=1 Ohm  i_specify=off  i_priority=None  i=0 A  i_nominal_specify=off  i_nominal_unit=A  i_nominal_value=1  v_specify=off  v_priority=None  v=0 V  v_nominal_specify=off  v_nominal_unit=V  v_nominal_value=1
  Resistor2 : fl_lib/Electrical/Electrical Elements/Resistor  R=1 Ohm  i_specify=off  i_priority=None  i=0 A  i_nominal_specify=off  i_nominal_unit=A  i_nominal_value=1  v_specify=off  v_priority=None  v=0 V  v_nominal_specify=off  v_nominal_unit=V  v_nominal_value=1
  Sensor dynamics : Subsystem
  ABC1 : PMIOPort  Side=Left
  ABC2 : PMIOPort  Port=2  Side=Right
  Out1 : Outport
  wires:
  PS-Simulink Converter1/1 -> Sensor dynamics/1(V)
  Sensor dynamics/1(I) -> Out1/1
  connections:
  Phase Splitter/LConn1 -- ABC1/RConn1
  ABC2/RConn1 -- Phase Splitter1/LConn1
  Connection Label19/LConn1 -- Phase Voltage Sensor (Three-Phase)1/LConn3
  Connection Label18/LConn1 -- Phase Voltage Sensor (Three-Phase)1/LConn2
  PS-Simulink Converter1/LConn1 -- Phase Voltage Sensor (Three-Phase)1/RConn1
  Connection Label20/LConn1 -- Phase Voltage Sensor (Three-Phase)1/LConn1
  Nonlinear Transformer/RConn1 -- Resistor/LConn1 -- Connection Label12/LConn1
  Nonlinear Transformer/LConn1 -- Phase Splitter/RConn1
  Phase Splitter1/RConn1 -- Nonlinear Transformer/LConn2
  Resistor/RConn1 -- Connection Label1/LConn1 -- Nonlinear Transformer/RConn2
  Nonlinear Transformer1/RConn1 -- Resistor1/LConn1 -- Connection Label3/LConn1
  Nonlinear Transformer1/LConn2 -- Phase Splitter1/RConn2
  Nonlinear Transformer1/LConn1 -- Phase Splitter/RConn2
  Nonlinear Transformer2/RConn1 -- Resistor2/LConn1 -- Connection Label8/LConn1
  Nonlinear Transformer2/LConn1 -- Phase Splitter/RConn3
  Phase Splitter1/RConn3 -- Nonlinear Transformer2/LConn2
  Resistor2/RConn1 -- Connection Label4/LConn1 -- Nonlinear Transformer2/RConn2
  Resistor1/RConn1 -- Nonlinear Transformer1/RConn2 -- Connection Label2/LConn1
  Electrical Reference/LConn1 -- Phase Voltage Sensor (Three-Phase)1/RConn2 -- Phase Voltage Sensor (Three-Phase)1/RConn3 -- Phase Voltage Sensor (Three-Phase)1/RConn4
  Connection Label5/LConn1 -- Grounded Neutral (Three-Phase)1/LConn1
  Connection Label6/LConn1 -- Grounded Neutral (Three-Phase)1/LConn2
  Connection Label7/LConn1 -- Grounded Neutral (Three-Phase)1/LConn3

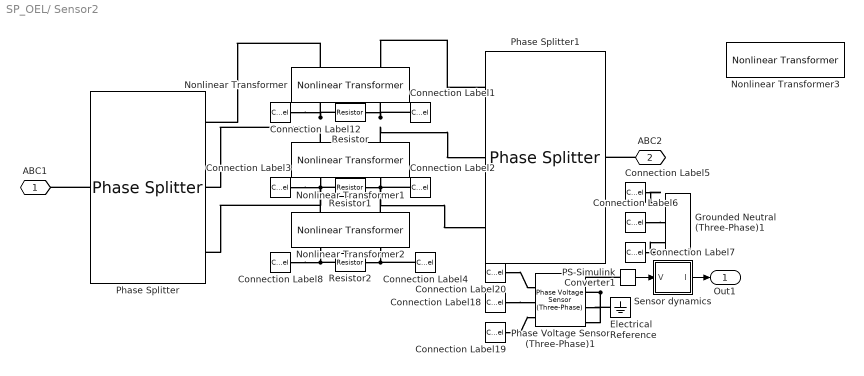
== system SP_OEL/ Sensor2 ==
  Connection Label1 : ConnectionLabel  Label=Ian
  Connection Label12 : ConnectionLabel  Label=Iap
  Connection Label18 : ConnectionLabel  Label=Ibp
  Connection Label19 : ConnectionLabel  Label=Icp
  Connection Label2 : ConnectionLabel  Label=Ibn
  Connection Label20 : ConnectionLabel  Label=Iap
  Connection Label3 : ConnectionLabel  Label=Ibp
  Connection Label4 : ConnectionLabel  Label=Ibn
  Connection Label5 : ConnectionLabel  Label=Ian
  Connection Label6 : ConnectionLabel  Label=Ibn
  Connection Label7 : ConnectionLabel  Label=Icn
  Connection Label8 : ConnectionLabel  Label=Icp
  Electrical Reference : fl_lib/Electrical/Electrical Elements/Electrical Reference
  Grounded Neutral (Three-Phase)1 : ee_lib/Connectors & References/Grounded Neutral (Three-Phase)
      settings: InternalSimscapePortConfiguration="{\"Bottom\":[],\"Left\":[{\"id\":\"a\",\"label\":\"a\",\"type\":\"foundation.electrical.electrical\"},{\"id\":\"b\",\"label\":\"b\",\"type\":\"foundation.electrical.electrical\"},{\"id\":\"c\",\"label\":\"c\",\"type\":\"foundation.electrical.electrical\"}],\"Right\":[],\"Top\":[]}"
  Nonlinear Transformer : ee_lib/Passive/Transformers/Nonlinear Transformer  Nw=1  Nw2=500  winding_param_option=1  Req=1e-3 Ohm  Leq=1e-4 H  R_1=0.01 Ohm  L_1=0.0001 H  R_2=0.01 Ohm  L_2=0.0001 H  averaging_period=0 s  R_m=100 Ohm  parameterization_option=1  H_data=[0, 200, 400, 600, 800, 1000] A/m  B_data=[0, .81, 1.25, 1.42, 1.48, 1.49] T  length_effective=0.2 m  area_effective=2e-4 m^2  L=4e-2 H  L_sat=1e-2 H  current_data=[0, .4, .8, 1.2, 1.6, 2] A  magnetic_flux_data=[0, .161, .25, .284, .295, .299] .* 1e-3 Wb  magnetic_flux_sat=1.6e-04 Wb  dBdH0=0.005 m*T/A  B1=1.49 T  H1=1000 A/m  c=0.1  K=200 A/m  alpha=1e-4  interpolation_option=1  Leq_i0=0 A  L1_i0=0 A  L2_i0=0 A  x0_option=1  i_L0=0 A  phi0=0 Wb  B0=0 T  H0=0 A/m  Leq_g=1e-9 1/Ohm  L1_g=1e-9 1/Ohm  L2_g=1e-9 1/Ohm
      settings: InternalSimscapePortConfiguration="{\"Bottom\":[],\"Left\":[{\"id\":\"p1\",\"label\":\"1+\",\"type\":\"foundation.electrical.electrical\"},{\"id\":\"n1\",\"label\":\"1-\",\"type\":\"foundation.electrical.electrical\"}],\"Right\":[{\"id\":\"p2\",\"label\":\"2+\",\"type\":\"foundation.electrical.electrical\"},{\"id\":\"n2\",\"label\":\"2-\",\"type\":\"foundation.electrical.electrical\"}],\"Top\":[]}"
  Nonlinear Transformer1 : ee_lib/Passive/Transformers/Nonlinear Transformer  Nw=1  Nw2=500  winding_param_option=1  Req=1e-3 Ohm  Leq=1e-4 H  R_1=0.01 Ohm  L_1=0.0001 H  R_2=0.01 Ohm  L_2=0.0001 H  averaging_period=0 s  R_m=100 Ohm  parameterization_option=1  H_data=[0, 200, 400, 600, 800, 1000] A/m  B_data=[0, .81, 1.25, 1.42, 1.48, 1.49] T  length_effective=0.2 m  area_effective=2e-4 m^2  L=4e-2 H  L_sat=1e-2 H  current_data=[0, .4, .8, 1.2, 1.6, 2] A  magnetic_flux_data=[0, .161, .25, .284, .295, .299] .* 1e-3 Wb  magnetic_flux_sat=1.6e-04 Wb  dBdH0=0.005 m*T/A  B1=1.49 T  H1=1000 A/m  c=0.1  K=200 A/m  alpha=1e-4  interpolation_option=1  Leq_i0=0 A  L1_i0=0 A  L2_i0=0 A  x0_option=1  i_L0=0 A  phi0=0 Wb  B0=0 T  H0=0 A/m  Leq_g=1e-9 1/Ohm  L1_g=1e-9 1/Ohm  L2_g=1e-9 1/Ohm
      settings: InternalSimscapePortConfiguration="{\"Bottom\":[],\"Left\":[{\"id\":\"p1\",\"label\":\"1+\",\"type\":\"foundation.electrical.electrical\"},{\"id\":\"n1\",\"label\":\"1-\",\"type\":\"foundation.electrical.electrical\"}],\"Right\":[{\"id\":\"p2\",\"label\":\"2+\",\"type\":\"foundation.electrical.electrical\"},{\"id\":\"n2\",\"label\":\"2-\",\"type\":\"foundation.electrical.electrical\"}],\"Top\":[]}"
  Nonlinear Transformer2 : ee_lib/Passive/Transformers/Nonlinear Transformer  Nw=1  Nw2=500  winding_param_option=1  Req=1e-3 Ohm  Leq=1e-4 H  R_1=0.01 Ohm  L_1=0.0001 H  R_2=0.01 Ohm  L_2=0.0001 H  averaging_period=0 s  R_m=100 Ohm  parameterization_option=1  H_data=[0, 200, 400, 600, 800, 1000] A/m  B_data=[0, .81, 1.25, 1.42, 1.48, 1.49] T  length_effective=0.2 m  area_effective=2e-4 m^2  L=4e-2 H  L_sat=1e-2 H  current_data=[0, .4, .8, 1.2, 1.6, 2] A  magnetic_flux_data=[0, .161, .25, .284, .295, .299] .* 1e-3 Wb  magnetic_flux_sat=1.6e-04 Wb  dBdH0=0.005 m*T/A  B1=1.49 T  H1=1000 A/m  c=0.1  K=200 A/m  alpha=1e-4  interpolation_option=1  Leq_i0=0 A  L1_i0=0 A  L2_i0=0 A  x0_option=1  i_L0=0 A  phi0=0 Wb  B0=0 T  H0=0 A/m  Leq_g=1e-9 1/Ohm  L1_g=1e-9 1/Ohm  L2_g=1e-9 1/Ohm
      settings: InternalSimscapePortConfiguration="{\"Bottom\":[],\"Left\":[{\"id\":\"p1\",\"label\":\"1+\",\"type\":\"foundation.electrical.electrical\"},{\"id\":\"n1\",\"label\":\"1-\",\"type\":\"foundation.electrical.electrical\"}],\"Right\":[{\"id\":\"p2\",\"label\":\"2+\",\"type\":\"foundation.electrical.electrical\"},{\"id\":\"n2\",\"label\":\"2-\",\"type\":\"foundation.electrical.electrical\"}],\"Top\":[]}"
  Nonlinear Transformer3 : ee_lib/Passive/Transformers/Nonlinear Transformer  Nw=1  Nw2=sensor2.ctRatio  winding_param_option=1  Req=1e-3 Ohm  Leq=1e-4 H  R_1=0.01 Ohm  L_1=0.0001 H  R_2=0.01 Ohm  L_2=0.0001 H  averaging_period=0 s  R_m=100 Ohm  parameterization_option=1  H_data=[0, 200, 400, 600, 800, 1000] A/m  B_data=[0, .81, 1.25, 1.42, 1.48, 1.49] T  length_effective=0.2 m  area_effective=2e-4 m^2  L=4e-2 H  L_sat=1e-2 H  current_data=[0, .4, .8, 1.2, 1.6, 2] A  magnetic_flux_data=[0, .161, .25, .284, .295, .299] .* 1e-3 Wb  magnetic_flux_sat=1.6e-04 Wb  dBdH0=0.005 m*T/A  B1=1.49 T  H1=1000 A/m  c=0.1  K=200 A/m  alpha=1e-4  interpolation_option=1  Leq_i0=0 A  L1_i0=0 A  L2_i0=0 A  x0_option=1  i_L0=0 A  phi0=0 Wb  B0=0 T  H0=0 A/m  Leq_g=1e-9 1/Ohm  L1_g=1e-9 1/Ohm  L2_g=1e-9 1/Ohm
      settings: InternalSimscapePortConfiguration="{\"Bottom\":[],\"Left\":[{\"id\":\"p1\",\"label\":\"1+\",\"type\":\"foundation.electrical.electrical\"},{\"id\":\"n1\",\"label\":\"1-\",\"type\":\"foundation.electrical.electrical\"}],\"Right\":[{\"id\":\"p2\",\"label\":\"2+\",\"type\":\"foundation.electrical.electrical\"},{\"id\":\"n2\",\"label\":\"2-\",\"type\":\"foundation.electrical.electrical\"}],\"Top\":[]}"
  PS-Simulink Converter1 : nesl_utility/PS-Simulink Converter  PhysicalDomain=network_engine_domain  SubClassName=ps_output  LeftPortType=input  RightPortType=output  PseudoPeriodic=off  Frequencies=[]  VectorFormat=1-D array  Unit=inherit  AffineConversion=off
  Phase Splitter : ee_lib/Connectors & References/Phase Splitter
  Phase Splitter1 : ee_lib/Connectors & References/Phase Splitter
  Phase Voltage Sensor (Three-Phase)1 : ee_lib/Sensors & Transducers/Phase Voltage Sensor (Three-Phase)
      settings: LogSimulationData=on  InternalSimscapePortConfiguration="{\"Bottom\":[],\"Left\":[{\"id\":\"a1\",\"label\":\"a1\",\"type\":\"foundation.electrical.electrical\"},{\"id\":\"b1\",\"label\":\"b1\",\"type\":\"foundation.electrical.electrical\"},{\"id\":\"c1\",\"label\":\"c1\",\"type\":\"foundation.electrical.electrical\"}],\"Right\":[{\"id\":\"V_output\",\"label\":\"V\",\"type\":\"output\"},{\"id\":\"a2\",\"label\":\"a2\",\"type\":\"foundation.electrical.electrical\"},{\"id\":\"b2\",\"label\":\"b2\",\"type\":\"foundation.electrical.electrical\"},{\"id\":\"c2\",\"label\":\"c2\",\"type\":\"foundation.electrical.electrical\"}],\"Top\":[]}"
  Resistor : fl_lib/Electrical/Electrical Elements/Resistor  R=1 Ohm  i_specify=off  i_priority=None  i=0 A  i_nominal_specify=off  i_nominal_unit=A  i_nominal_value=1  v_specify=off  v_priority=None  v=0 V  v_nominal_specify=off  v_nominal_unit=V  v_nominal_value=1
  Resistor1 : fl_lib/Electrical/Electrical Elements/Resistor  R=1 Ohm  i_specify=off  i_priority=None  i=0 A  i_nominal_specify=off  i_nominal_unit=A  i_nominal_value=1  v_specify=off  v_priority=None  v=0 V  v_nominal_specify=off  v_nominal_unit=V  v_nominal_value=1
  Resistor2 : fl_lib/Electrical/Electrical Elements/Resistor  R=1 Ohm  i_specify=off  i_priority=None  i=0 A  i_nominal_specify=off  i_nominal_unit=A  i_nominal_value=1  v_specify=off  v_priority=None  v=0 V  v_nominal_specify=off  v_nominal_unit=V  v_nominal_value=1
  Sensor dynamics : Subsystem
  ABC1 : PMIOPort  Side=Left
  ABC2 : PMIOPort  Port=2  Side=Right
  Out1 : Outport
  wires:
  PS-Simulink Converter1/1 -> Sensor dynamics/1(V)
  Sensor dynamics/1(I) -> Out1/1
  connections:
  Phase Splitter/LConn1 -- ABC1/RConn1
  ABC2/RConn1 -- Phase Splitter1/LConn1
  Connection Label19/LConn1 -- Phase Voltage Sensor (Three-Phase)1/LConn3
  Connection Label18/LConn1 -- Phase Voltage Sensor (Three-Phase)1/LConn2
  PS-Simulink Converter1/LConn1 -- Phase Voltage Sensor (Three-Phase)1/RConn1
  Connection Label20/LConn1 -- Phase Voltage Sensor (Three-Phase)1/LConn1
  Nonlinear Transformer/RConn1 -- Resistor/LConn1 -- Connection Label12/LConn1
  Nonlinear Transformer/LConn1 -- Phase Splitter/RConn1
  Phase Splitter1/RConn1 -- Nonlinear Transformer/LConn2
  Nonlinear Transformer/RConn2 -- Resistor/RConn1 -- Connection Label1/LConn1
  Resistor1/LConn1 -- Nonlinear Transformer1/RConn1 -- Connection Label3/LConn1
  Nonlinear Transformer1/LConn2 -- Phase Splitter1/RConn2
  Nonlinear Transformer1/LConn1 -- Phase Splitter/RConn2
  Resistor2/LConn1 -- Nonlinear Transformer2/RConn1 -- Connection Label8/LConn1
  Nonlinear Transformer2/LConn1 -- Phase Splitter/RConn3
  Nonlinear Transformer2/LConn2 -- Phase Splitter1/RConn3
  Resistor2/RConn1 -- Nonlinear Transformer2/RConn2 -- Connection Label4/LConn1
  Connection Label2/LConn1 -- Nonlinear Transformer1/RConn2 -- Resistor1/RConn1
  Phase Voltage Sensor (Three-Phase)1/RConn2 -- Phase Voltage Sensor (Three-Phase)1/RConn3 -- Electrical Reference/LConn1 -- Phase Voltage Sensor (Three-Phase)1/RConn4
  Connection Label5/LConn1 -- Grounded Neutral (Three-Phase)1/LConn1
  Connection Label6/LConn1 -- Grounded Neutral (Three-Phase)1/LConn2
  Connection Label7/LConn1 -- Grounded Neutral (Three-Phase)1/LConn3

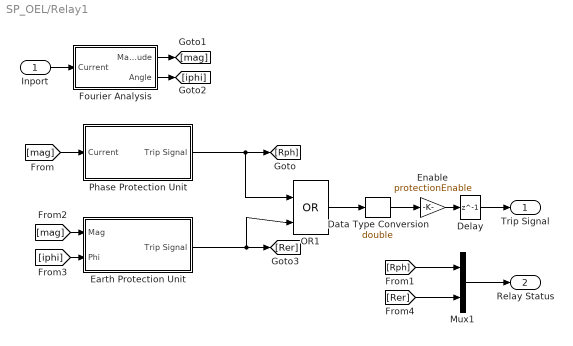
== system SP_OEL/Relay1 ==
  Inport : Inport
  Data Type Conversion : DataTypeConversion  OutDataTypeStr=double  SaturateOnIntegerOverflow=off  RndMeth=Floor
  Delay : Delay  DelayLength=1
  Earth Protection Unit : Subsystem
  Enable : Gain  Gain=protectionEnable
  Fourier Analysis : Subsystem
  Mux1 : Mux  Inputs=2
  OR1 : Logic  Operator=OR  IconShape=distinctive  AllPortsSameDT=off  OutDataTypeStr=boolean
  Phase Protection Unit : Subsystem
  Trip Signal : Outport
  Relay Status : Outport  Port=2
  wires:
  Data Type Conversion/1 -> Enable/1
  Enable/1 -> Delay/1
  Delay/1 -> Trip Signal/1
  [Rer] -> Mux1/2
  [Rph] -> Mux1/1
  Mux1/1 -> Relay Status/1
  OR1/1 -> Data Type Conversion/1
  Inport/1 -> Fourier Analysis/1(Current)
  Fourier Analysis/1(Magnitude) -> [mag]
  Fourier Analysis/2(Angle) -> [iphi]
  [mag] -> Phase Protection Unit/1(Current)
  [mag] -> Earth Protection Unit/1(Mag)
  [iphi] -> Earth Protection Unit/2(Phi)
  Phase Protection Unit/1(Trip Signal) -> OR1/1, [Rph]
  Earth Protection Unit/1(Trip Signal) -> [Rer], OR1/2

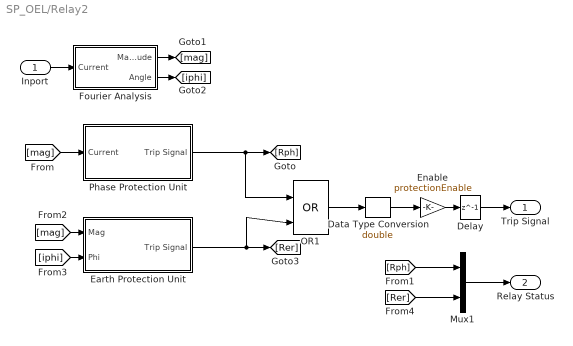
== system SP_OEL/Relay2 ==
  Inport : Inport
  Data Type Conversion : DataTypeConversion  OutDataTypeStr=double  SaturateOnIntegerOverflow=off  RndMeth=Floor
  Delay : Delay  DelayLength=1
  Earth Protection Unit : Subsystem
  Enable : Gain  Gain=protectionEnable
  Fourier Analysis : Subsystem
  Mux1 : Mux  Inputs=2
  OR1 : Logic  Operator=OR  IconShape=distinctive  AllPortsSameDT=off  OutDataTypeStr=boolean
  Phase Protection Unit : Subsystem
  Trip Signal : Outport
  Relay Status : Outport  Port=2
  wires:
  Data Type Conversion/1 -> Enable/1
  Enable/1 -> Delay/1
  Delay/1 -> Trip Signal/1
  [Rer] -> Mux1/2
  [Rph] -> Mux1/1
  Mux1/1 -> Relay Status/1
  OR1/1 -> Data Type Conversion/1
  Inport/1 -> Fourier Analysis/1(Current)
  Fourier Analysis/1(Magnitude) -> [mag]
  Fourier Analysis/2(Angle) -> [iphi]
  [mag] -> Phase Protection Unit/1(Current)
  [mag] -> Earth Protection Unit/1(Mag)
  [iphi] -> Earth Protection Unit/2(Phi)
  Phase Protection Unit/1(Trip Signal) -> OR1/1, [Rph]
  Earth Protection Unit/1(Trip Signal) -> [Rer], OR1/2
